simulink model "test_interconnect"  (Simulink 7.3)
settings: Solver=ode45  StartTime=0.0  StopTime=100  RelTol=1e-3
undefined symbols (not defined in the file): ROACH
libraries: xbsIndex_r4 x68, isi_correlator_lib x16, xps_library x7, casper_library x1
settings Model: Creator=wjm  LastModifiedBy=wjm
settings OptimizationCC: InitFltsAndDblsToZero=on

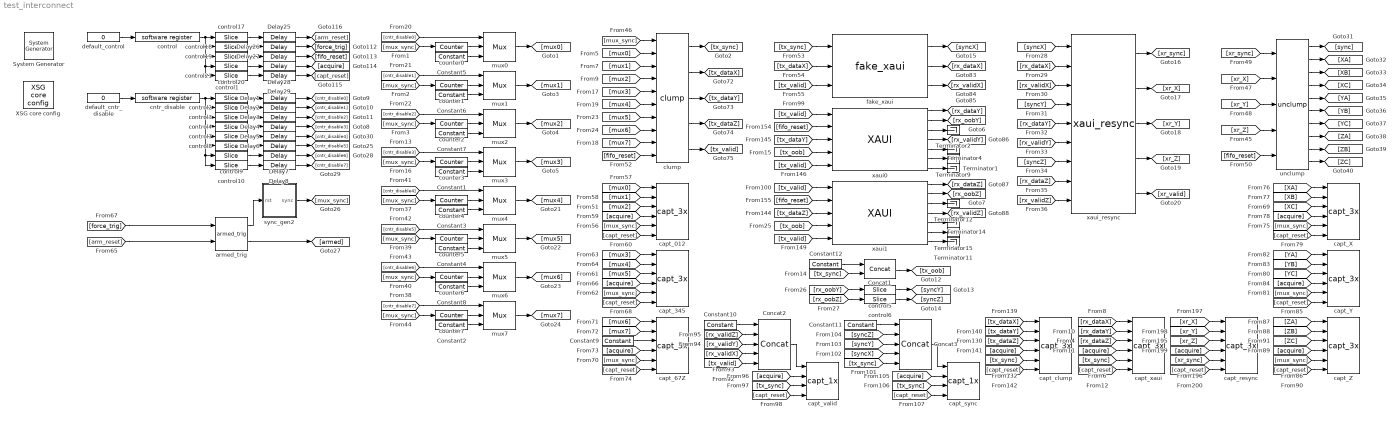
== system test_interconnect ==
  " System Generator" : xbsIndex_r4/ System Generator  Tag=genX  SystemSampleTime=-1  xilinxfamily=virtex5  part=xc5vsx95t  speed=-1  package=ff1136  synthesis_tool=XST  clock_wrapper=Clock Enables  directory=./test_interconnect/sysgen  testbench=off  simulink_period=1  sysclk_period=5  dcm_input_clock_period=100  incr_netlist=off  trim_vbits=Everywhere in SubSystem  dbl_ovrd=According to Block Masks  core_generation=According to Block Masks  run_coregen=off  deprecated_control=off  eval_field=0  block_type=sysgen
      settings: block_version=10.1.1
  Concat1 : xbsIndex_r4/Concat  num_inputs=2  dbl_ovrd=off  block_type=concat
      settings: block_version=11.3
  Concat2 : xbsIndex_r4/Concat  num_inputs=5  dbl_ovrd=off  block_type=concat
      settings: block_version=11.3
  Concat3 : xbsIndex_r4/Concat  num_inputs=5  dbl_ovrd=off  block_type=concat
      settings: block_version=11.3
  Constant{1..9} (9 alike) : xbsIndex_r4/Constant  arith_type=Unsigned  const=0  n_bits=8  bin_pt=0  explicit_period=on  period=1  equ=P=C  opselect=C  inp2=PCIN>>17  opr=+  inp1=P  carry=CIN  dbl_ovrd=off  block_type=constant
      settings: block_version=10.1.1
  Constant10 : xbsIndex_r4/Constant  arith_type=Unsigned  const=0  n_bits=28  bin_pt=0  explicit_period=on  period=1  equ=P=C  opselect=C  inp2=PCIN>>17  opr=+  inp1=P  carry=CIN  dbl_ovrd=off  block_type=constant
      settings: block_version=10.1.1
  Constant11 : xbsIndex_r4/Constant  arith_type=Unsigned  const=0  n_bits=28  bin_pt=0  explicit_period=on  period=1  equ=P=C  opselect=C  inp2=PCIN>>17  opr=+  inp1=P  carry=CIN  dbl_ovrd=off  block_type=constant
      settings: block_version=10.1.1
  Constant12 : xbsIndex_r4/Constant  arith_type=Unsigned  const=0  n_bits=3  bin_pt=0  explicit_period=on  period=1  equ=P=C  opselect=C  inp2=PCIN>>17  opr=+  inp1=P  carry=CIN  dbl_ovrd=off  block_type=constant
      settings: block_version=10.1.1
  Delay{1..8,25..29} (13 alike) : xbsIndex_r4/Delay  en=off  latency=3  dbl_ovrd=off  reg_retiming=off  block_type=delay
  Terminator{1..2,4,9,11..12,14..15} (8 alike) : Terminator
  XSG core config : xps_library/XSG core config  Tag=xps:xsg  SystemSampleTime=-1  hw_sys=ROACH:sx95t  ibob_linux=off  clk_src=sys_clk2x  iBOB_clk_src=sys_clk  BEE2_ctrl_clk_src=sys_clk  BEE2_usr_clk_src=sys_clk  ROACH_clk_src=sys_clk2x  CORR_clk_src=sys_clk  gpio_clk_io_group=iBOB:sma  gpio_clk_bit_index=0  clk_rate=200  sample_period=1  synthesis_tool=XST  mpc_type=powerpc440_ext
  armed_trig : isi_correlator_lib/armed_trig  SystemSampleTime=-1
  capt_012 : isi_correlator_lib/capt_3x  SystemSampleTime=-1
      link override bram0/convert_din: arith_type=Unsigned
      link override bram0/mem/sim_data_in: arith_type=Unsigned
      link override bram0/test_link_mux_demux_capt_demux_bram0_data_out: arith_type=Unsigned
      link override bram1/convert_din: arith_type=Unsigned
      link override bram1/mem/sim_data_in: arith_type=Unsigned
      link override bram1/test_link_mux_demux_capt_demux_bram1_data_out: arith_type=Unsigned
      link override bram2/convert_din: arith_type=Unsigned
      link override bram2/mem/sim_data_in: arith_type=Unsigned
      link override bram2/test_link_mux_demux_capt_demux_bram2_data_out: arith_type=Unsigned
  capt_345 : isi_correlator_lib/capt_3x  SystemSampleTime=-1
      link override bram0/convert_din: arith_type=Unsigned
      link override bram0/mem/sim_data_in: arith_type=Unsigned
      link override bram0/test_link_mux_demux_capt_demux_bram0_data_out: arith_type=Unsigned
      link override bram1/convert_din: arith_type=Unsigned
      link override bram1/mem/sim_data_in: arith_type=Unsigned
      link override bram1/test_link_mux_demux_capt_demux_bram1_data_out: arith_type=Unsigned
      link override bram2/convert_din: arith_type=Unsigned
      link override bram2/mem/sim_data_in: arith_type=Unsigned
      link override bram2/test_link_mux_demux_capt_demux_bram2_data_out: arith_type=Unsigned
  capt_67Z : isi_correlator_lib/capt_3x  SystemSampleTime=-1
      link override bram0/convert_din: arith_type=Unsigned
      link override bram0/mem/sim_data_in: arith_type=Unsigned
      link override bram0/test_link_mux_demux_capt_demux_bram0_data_out: arith_type=Unsigned
      link override bram1/convert_din: arith_type=Unsigned
      link override bram1/mem/sim_data_in: arith_type=Unsigned
      link override bram1/test_link_mux_demux_capt_demux_bram1_data_out: arith_type=Unsigned
      link override bram2/convert_din: arith_type=Unsigned
      link override bram2/mem/sim_data_in: arith_type=Unsigned
      link override bram2/test_link_mux_demux_capt_demux_bram2_data_out: arith_type=Unsigned
  capt_X : isi_correlator_lib/capt_3x  SystemSampleTime=-1
      link override bram0/convert_din: arith_type=Unsigned
      link override bram0/mem/sim_data_in: arith_type=Unsigned
      link override bram0/test_link_mux_demux_capt_demux_bram0_data_out: arith_type=Unsigned
      link override bram1/convert_din: arith_type=Unsigned
      link override bram1/mem/sim_data_in: arith_type=Unsigned
      link override bram1/test_link_mux_demux_capt_demux_bram1_data_out: arith_type=Unsigned
      link override bram2/convert_din: arith_type=Unsigned
      link override bram2/mem/sim_data_in: arith_type=Unsigned
      link override bram2/test_link_mux_demux_capt_demux_bram2_data_out: arith_type=Unsigned
  capt_Y : isi_correlator_lib/capt_3x  SystemSampleTime=-1
      link override bram0/convert_din: arith_type=Unsigned
      link override bram0/mem/sim_data_in: arith_type=Unsigned
      link override bram0/test_link_mux_demux_capt_demux_bram0_data_out: arith_type=Unsigned
      link override bram1/convert_din: arith_type=Unsigned
      link override bram1/mem/sim_data_in: arith_type=Unsigned
      link override bram1/test_link_mux_demux_capt_demux_bram1_data_out: arith_type=Unsigned
      link override bram2/convert_din: arith_type=Unsigned
      link override bram2/mem/sim_data_in: arith_type=Unsigned
      link override bram2/test_link_mux_demux_capt_demux_bram2_data_out: arith_type=Unsigned
  capt_Z : isi_correlator_lib/capt_3x  SystemSampleTime=-1
      link override bram0/convert_din: arith_type=Unsigned
      link override bram0/mem/sim_data_in: arith_type=Unsigned
      link override bram0/test_link_mux_demux_capt_demux_bram0_data_out: arith_type=Unsigned
      link override bram1/convert_din: arith_type=Unsigned
      link override bram1/mem/sim_data_in: arith_type=Unsigned
      link override bram1/test_link_mux_demux_capt_demux_bram1_data_out: arith_type=Unsigned
      link override bram2/convert_din: arith_type=Unsigned
      link override bram2/mem/sim_data_in: arith_type=Unsigned
      link override bram2/test_link_mux_demux_capt_demux_bram2_data_out: arith_type=Unsigned
  capt_clump : isi_correlator_lib/capt_3x  SystemSampleTime=-1
  capt_resync : isi_correlator_lib/capt_3x  SystemSampleTime=-1
      link override bram0/convert_din: arith_type=Unsigned
      link override bram0/mem/sim_data_in: arith_type=Unsigned
      link override bram0/test_link_mux_demux_capt_demux_bram0_data_out: arith_type=Unsigned
      link override bram1/convert_din: arith_type=Unsigned
      link override bram1/mem/sim_data_in: arith_type=Unsigned
      link override bram1/test_link_mux_demux_capt_demux_bram1_data_out: arith_type=Unsigned
      link override bram2/convert_din: arith_type=Unsigned
      link override bram2/mem/sim_data_in: arith_type=Unsigned
      link override bram2/test_link_mux_demux_capt_demux_bram2_data_out: arith_type=Unsigned
  capt_sync : isi_correlator_lib/capt_1x  SystemSampleTime=-1
  capt_valid : isi_correlator_lib/capt_1x  SystemSampleTime=-1
  capt_xaui : isi_correlator_lib/capt_3x  SystemSampleTime=-1
      link override bram0/convert_din: arith_type=Unsigned
      link override bram0/mem/sim_data_in: arith_type=Unsigned
      link override bram0/test_link_mux_demux_capt_demux_bram0_data_out: arith_type=Unsigned
      link override bram1/convert_din: arith_type=Unsigned
      link override bram1/mem/sim_data_in: arith_type=Unsigned
      link override bram1/test_link_mux_demux_capt_demux_bram1_data_out: arith_type=Unsigned
      link override bram2/convert_din: arith_type=Unsigned
      link override bram2/mem/sim_data_in: arith_type=Unsigned
      link override bram2/test_link_mux_demux_capt_demux_bram2_data_out: arith_type=Unsigned
  clump : isi_correlator_lib/clump  SystemSampleTime=-1  latency=1
  cntr_disable : xps_library/software register  Tag=xps:sw_reg  SystemSampleTime=-1  io_dir=From Processor  arith_type=Unsigned  bitwidth=32  bin_pt=0  sample_period=1  gw_name=test_interconnect_cntr_disable_user_data_out
      link override corr_3ghz_10_1_corr_id_user_data_out: arith_type=Unsigned  n_bits=32  bin_pt=0  period=1
      link override corr_3ghz_10_1_exp_corr_id_user_data_out: arith_type=Unsigned  n_bits=32  bin_pt=0  period=1
      link override isi_corr_eq_coeff_user_data_out: arith_type=Unsigned  n_bits=32  bin_pt=0  period=1
      link override isi_correlator_control_user_data_out: arith_type=Unsigned  n_bits=32  bin_pt=0  period=1
      link override isi_correlator_cropped_control_user_data_out: arith_type=Unsigned  n_bits=32  bin_pt=0  period=1
      link override isi_correlator_eq_coeff_user_data_out: arith_type=Unsigned  n_bits=32  bin_pt=0  period=1
      link override isi_spectrometer_control_user_data_out: arith_type=Unsigned  n_bits=32  bin_pt=0  period=1
      link override isi_spectrometer_cropped_control_user_data_out: arith_type=Unsigned  n_bits=32  bin_pt=0  period=1
      link override isi_spectrometer_with_pfb_control_user_data_out: arith_type=Unsigned  n_bits=32  bin_pt=0  period=1
      link override roach_spectrometer_control_user_data_out: arith_type=Unsigned  n_bits=32  bin_pt=0  period=1
      link override test_link_mux_demux_control_user_data_out: arith_type=Unsigned  n_bits=32  bin_pt=0  period=1
  control : xps_library/software register  Tag=xps:sw_reg  SystemSampleTime=-1  io_dir=From Processor  arith_type=Unsigned  bitwidth=32  bin_pt=0  sample_period=1  gw_name=test_interconnect_control_user_data_out
      link override corr_3ghz_10_1_corr_id_user_data_out: arith_type=Unsigned  n_bits=32  bin_pt=0  period=1
      link override corr_3ghz_10_1_exp_corr_id_user_data_out: arith_type=Unsigned  n_bits=32  bin_pt=0  period=1
      link override isi_corr_eq_coeff_user_data_out: arith_type=Unsigned  n_bits=32  bin_pt=0  period=1
      link override isi_correlator_control_user_data_out: arith_type=Unsigned  n_bits=32  bin_pt=0  period=1
      link override isi_correlator_cropped_control_user_data_out: arith_type=Unsigned  n_bits=32  bin_pt=0  period=1
      link override isi_correlator_eq_coeff_user_data_out: arith_type=Unsigned  n_bits=32  bin_pt=0  period=1
      link override isi_spectrometer_control_user_data_out: arith_type=Unsigned  n_bits=32  bin_pt=0  period=1
      link override isi_spectrometer_cropped_control_user_data_out: arith_type=Unsigned  n_bits=32  bin_pt=0  period=1
      link override isi_spectrometer_with_pfb_control_user_data_out: arith_type=Unsigned  n_bits=32  bin_pt=0  period=1
      link override roach_spectrometer_control_user_data_out: arith_type=Unsigned  n_bits=32  bin_pt=0  period=1
      link override test_link_mux_demux_control_user_data_out: arith_type=Unsigned  n_bits=32  bin_pt=0  period=1
  control1 : xbsIndex_r4/Slice  nbits=1  boolean_output=off  mode=Lower Bit Location + Width  bit1=0  base1=MSB of Input  bit0=0  base0=LSB of Input  dbl_ovrd=off  block_type=slice
      settings: block_version=10.1.3
  control10 : xbsIndex_r4/Slice  nbits=1  boolean_output=off  mode=Lower Bit Location + Width  bit1=0  base1=MSB of Input  bit0=7  base0=LSB of Input  dbl_ovrd=off  block_type=slice
      settings: block_version=10.1.3
  control17 : xbsIndex_r4/Slice  nbits=1  boolean_output=on  mode=Lower Bit Location + Width  bit1=0  base1=MSB of Input  bit0=0  base0=LSB of Input  dbl_ovrd=off  block_type=slice
      settings: infoedit="Extracts a given range of bits from each input sample and presents it at the output.  The output type is ordinarily unsigned with binary point at zero, but can be Boolean when the slice is one bit wide.<P><P>Hardware notes: In hardware this block costs nothing."  block_version=10.1.3
  control18 : xbsIndex_r4/Slice  nbits=1  boolean_output=on  mode=Lower Bit Location + Width  bit1=0  base1=MSB of Input  bit0=1  base0=LSB of Input  dbl_ovrd=off  block_type=slice
      settings: infoedit="Extracts a given range of bits from each input sample and presents it at the output.  The output type is ordinarily unsigned with binary point at zero, but can be Boolean when the slice is one bit wide.<P><P>Hardware notes: In hardware this block costs nothing."  block_version=10.1.3
  control19 : xbsIndex_r4/Slice  nbits=1  boolean_output=on  mode=Lower Bit Location + Width  bit1=0  base1=MSB of Input  bit0=2  base0=LSB of Input  dbl_ovrd=off  block_type=slice
      settings: infoedit="Extracts a given range of bits from each input sample and presents it at the output.  The output type is ordinarily unsigned with binary point at zero, but can be Boolean when the slice is one bit wide.<P><P>Hardware notes: In hardware this block costs nothing."  block_version=10.1.3
  control2 : xbsIndex_r4/Slice  nbits=1  boolean_output=off  mode=Lower Bit Location + Width  bit1=0  base1=MSB of Input  bit0=1  base0=LSB of Input  dbl_ovrd=off  block_type=slice
      settings: block_version=10.1.3
  control20 : xbsIndex_r4/Slice  nbits=1  boolean_output=on  mode=Lower Bit Location + Width  bit1=0  base1=MSB of Input  bit0=3  base0=LSB of Input  dbl_ovrd=off  block_type=slice
      settings: infoedit="Extracts a given range of bits from each input sample and presents it at the output.  The output type is ordinarily unsigned with binary point at zero, but can be Boolean when the slice is one bit wide.<P><P>Hardware notes: In hardware this block costs nothing."  block_version=10.1.3
  control21 : xbsIndex_r4/Slice  nbits=1  boolean_output=on  mode=Lower Bit Location + Width  bit1=0  base1=MSB of Input  bit0=4  base0=LSB of Input  dbl_ovrd=off  block_type=slice
      settings: infoedit="Extracts a given range of bits from each input sample and presents it at the output.  The output type is ordinarily unsigned with binary point at zero, but can be Boolean when the slice is one bit wide.<P><P>Hardware notes: In hardware this block costs nothing."  block_version=10.1.3
  control3 : xbsIndex_r4/Slice  nbits=1  boolean_output=off  mode=Lower Bit Location + Width  bit1=0  base1=MSB of Input  bit0=2  base0=LSB of Input  dbl_ovrd=off  block_type=slice
      settings: block_version=10.1.3
  control4 : xbsIndex_r4/Slice  nbits=1  boolean_output=off  mode=Lower Bit Location + Width  bit1=0  base1=MSB of Input  bit0=3  base0=LSB of Input  dbl_ovrd=off  block_type=slice
      settings: block_version=10.1.3
  control5 : xbsIndex_r4/Slice  nbits=1  boolean_output=on  mode=Lower Bit Location + Width  bit1=0  base1=MSB of Input  bit0=0  base0=LSB of Input  dbl_ovrd=off  block_type=slice
      settings: infoedit="Extracts a given range of bits from each input sample and presents it at the output.  The output type is ordinarily unsigned with binary point at zero, but can be Boolean when the slice is one bit wide.<P><P>Hardware notes: In hardware this block costs nothing."  block_version=10.1.3
  control6 : xbsIndex_r4/Slice  nbits=1  boolean_output=on  mode=Lower Bit Location + Width  bit1=0  base1=MSB of Input  bit0=0  base0=LSB of Input  dbl_ovrd=off  block_type=slice
      settings: infoedit="Extracts a given range of bits from each input sample and presents it at the output.  The output type is ordinarily unsigned with binary point at zero, but can be Boolean when the slice is one bit wide.<P><P>Hardware notes: In hardware this block costs nothing."  block_version=10.1.3
  control7 : xbsIndex_r4/Slice  nbits=1  boolean_output=off  mode=Lower Bit Location + Width  bit1=0  base1=MSB of Input  bit0=4  base0=LSB of Input  dbl_ovrd=off  block_type=slice
      settings: block_version=10.1.3
  control8 : xbsIndex_r4/Slice  nbits=1  boolean_output=off  mode=Lower Bit Location + Width  bit1=0  base1=MSB of Input  bit0=5  base0=LSB of Input  dbl_ovrd=off  block_type=slice
      settings: block_version=10.1.3
  control9 : xbsIndex_r4/Slice  nbits=1  boolean_output=off  mode=Lower Bit Location + Width  bit1=0  base1=MSB of Input  bit0=6  base0=LSB of Input  dbl_ovrd=off  block_type=slice
      settings: block_version=10.1.3
  counter0 : xbsIndex_r4/Counter  cnt_type=Free Running  cnt_to=Inf  operation=Up  start_count=0  cnt_by_val=128  arith_type=Unsigned  n_bits=8  bin_pt=0  load_pin=off  rst=on  en=off  explicit_period=on  period=1  dbl_ovrd=off  use_behavioral_HDL=off  implementation=Fabric  use_rpm=off  block_type=counter
  counter1 : xbsIndex_r4/Counter  cnt_type=Free Running  cnt_to=Inf  operation=Up  start_count=0  cnt_by_val=64  arith_type=Unsigned  n_bits=8  bin_pt=0  load_pin=off  rst=on  en=off  explicit_period=on  period=1  dbl_ovrd=off  use_behavioral_HDL=off  implementation=Fabric  use_rpm=off  block_type=counter
  counter2 : xbsIndex_r4/Counter  cnt_type=Free Running  cnt_to=Inf  operation=Up  start_count=0  cnt_by_val=32  arith_type=Unsigned  n_bits=8  bin_pt=0  load_pin=off  rst=on  en=off  explicit_period=on  period=1  dbl_ovrd=off  use_behavioral_HDL=off  implementation=Fabric  use_rpm=off  block_type=counter
  counter3 : xbsIndex_r4/Counter  cnt_type=Free Running  cnt_to=Inf  operation=Up  start_count=0  cnt_by_val=16  arith_type=Unsigned  n_bits=8  bin_pt=0  load_pin=off  rst=on  en=off  explicit_period=on  period=1  dbl_ovrd=off  use_behavioral_HDL=off  implementation=Fabric  use_rpm=off  block_type=counter
  counter4 : xbsIndex_r4/Counter  cnt_type=Free Running  cnt_to=Inf  operation=Up  start_count=0  cnt_by_val=8  arith_type=Unsigned  n_bits=8  bin_pt=0  load_pin=off  rst=on  en=off  explicit_period=on  period=1  dbl_ovrd=off  use_behavioral_HDL=off  implementation=Fabric  use_rpm=off  block_type=counter
  counter5 : xbsIndex_r4/Counter  cnt_type=Free Running  cnt_to=Inf  operation=Up  start_count=0  cnt_by_val=4  arith_type=Unsigned  n_bits=8  bin_pt=0  load_pin=off  rst=on  en=off  explicit_period=on  period=1  dbl_ovrd=off  use_behavioral_HDL=off  implementation=Fabric  use_rpm=off  block_type=counter
  counter6 : xbsIndex_r4/Counter  cnt_type=Free Running  cnt_to=Inf  operation=Up  start_count=0  cnt_by_val=2  arith_type=Unsigned  n_bits=8  bin_pt=0  load_pin=off  rst=on  en=off  explicit_period=on  period=1  dbl_ovrd=off  use_behavioral_HDL=off  implementation=Fabric  use_rpm=off  block_type=counter
  counter7 : xbsIndex_r4/Counter  cnt_type=Free Running  cnt_to=Inf  operation=Up  start_count=0  cnt_by_val=1  arith_type=Unsigned  n_bits=8  bin_pt=0  load_pin=off  rst=on  en=off  explicit_period=on  period=1  dbl_ovrd=off  use_behavioral_HDL=off  implementation=Fabric  use_rpm=off  block_type=counter
  default_cntr_disable : Constant  Value=0  OutDataType=sfix(16)  OutScaling=2^0  SampleTime=1
  default_control : Constant  Value=0  OutDataType=sfix(16)  OutScaling=2^0  SampleTime=1
  fake_xaui : isi_correlator_lib/fake_xaui  SystemSampleTime=-1  latency=32
  mux{0..7} (8 alike) : xbsIndex_r4/Mux  inputs=2  en=off  latency=0  precision=Full  arith_type=Unsigned  n_bits=16  bin_pt=14  quantization=Truncate  overflow=Wrap  dbl_ovrd=off  block_type=mux
      settings: block_version=11.3
  sync_gen2 : Subsystem  AncestorBlock=isi_correlator_lib/sync_gen2  mask(sync_gen2){using_pfb_fir=off, pfb_fir_taps=4, using_fft=off, fft_size=7, fft_inputs=4, fft_orders=[2 2 2 1], using_ct=off, ct_type=Double-buffered, using_vacc=off, vacc_length=0, using_scale_factor=on, scale_factor=2^10}
      mask prompts: using_pfb_fir "This design uses a PFB FIR."; pfb_fir_taps "Number of taps in PFB FIR:"; using_fft "This design uses an FFT."; fft_size "Size of FFT: (2^?)"; fft_inputs "Number of FFT inputs: (2^?)"; fft_orders "Order of FFT reorders: (vector)"; using_ct "This design uses a corner turner."; ct_type "Type of reorder operation:"; using_vacc "This design uses a vector accumulator."; vacc_length "Length of accumulations: (2^?)"; using_scale_factor "Scale the minimum period by an arbitrary amount."; scale_factor "Scale factor:"
      mask help: This block generates a sync pulse of an appropriate period based on the specified mask parameters.
      mask init:
      | sync_gen2_init(gcb, ...
      |     'using_pfb_fir', using_pfb_fir, ...
      |     'pfb_fir_taps', pfb_fir_taps, ...
      |     'using_fft', using_fft, ...
      |     'fft_size', fft_size, ...
      |     'fft_inputs', fft_inputs, ...
      |     'fft_orders', fft_orders, ...
      |     'using_ct', using_ct, ...
      |     'ct_type', ct_type, ...
      |     'using_vacc', using_vacc, ...
      |     'vacc_length', vacc_length, ...
      |     'using_scale_factor', using_scale_factor, ...
      |     'scale_factor', scale_factor);
      settings: AttributesFormatString=sync_period=1024
      mask StyleString: checkbox,edit,checkbox,edit,edit,edit,checkbox,popup(Double-buffered|In-place),checkbox,edit,checkbox,edit
      mask CallbackString:
      | thisVariable = 'using_pfb_fir';
      | affectedVars = {'pfb_fir_taps'};
      | 
      | thisBlock = gcb();
      | thisVarState = get_param(thisBlock, thisVariable);
      | maskNames = get_param(thisBlock, 'MaskNames');
      | maskEnables = get_param(thisBlock, 'MaskEnables');
      | 
      | for varName = affectedVars
      |     varIndex = find(ismember(maskNames, varName));
      |     maskEnables{varIndex} = thisVarState;
      | end
      | 
      | set_param(thisBlock, 'MaskEnables', maskEnables);||thisVariable = 'using_fft';
      | affectedVars = {'fft_size', 'fft_inputs', 'fft_orders'};
      | 
      | thisBlock = gcb();
      | thisVarState = get_param(thisBlock, thisVariable);
      | maskNames = get_param(thisBlock, 'MaskNames');
      | maskEnables = get_param(thisBlock, 'MaskEnables');
      | 
      | for varName = affectedVars
      |     varIndex = find(ismember(maskNames, varName));
      |     maskEnables{varIndex} = thisVarState;
      | end
      | 
      | set_param(thisBlock, 'MaskEnables', maskEnables);||||thisVariable = 'using_ct';
      | affectedVars = {'ct_type'};
      | 
      | thisBlock = gcb();
      | thisVarState = get_param(thisBlock, thisVariable);
      | maskNames = get_param(thisBlock, 'MaskNames');
      | maskEnables = get_param(thisBlock, 'MaskEnables');
      | 
      | for varName = affectedVars
      |     varIndex = find(ismember(maskNames, varName));
      |     maskEnables{varIndex} = thisVarState;
      | end
      | 
      | set_param(thisBlock, 'MaskEnables', maskEnables);||thisVariable = 'using_vacc';
      | affectedVars = {'vacc_length'};
      | 
      | thisBlock = gcb();
      | thisVarState = get_param(thisBlock, thisVariable);
      | maskNames = get_param(thisBlock, 'MaskNames');
      | maskEnables = get_param(thisBlock, 'MaskEnables');
      | 
      | for varName = affectedVars
      |     varIndex = find(ismember(maskNames, varName));
      |     maskEnables{varIndex} = thisVarState;
      | end
      | 
      | set_param(thisBlock, 'MaskEnables', maskEnables);||thisVariable = 'using_scale_factor';
      | affectedVars = {'scale_factor'};
      | 
      | thisBlock = gcb();
      | thisVarState = get_param(thisBlock, thisVariable);
      | maskNames = get_param(thisBlock, 'MaskNames');
      | maskEnables = get_param(thisBlock, 'MaskEnables');
      | 
      | for varName = affectedVars
      |     varIndex = find(ismember(maskNames, varName));
      |     maskEnables{varIndex} = thisVarState;
      | end
      | 
      | set_param(thisBlock, 'MaskEnables', maskEnables);|
  unclump : isi_correlator_lib/unclump  SystemSampleTime=-1  latency=1
  xaui0 : xps_library/XAUI  Tag=xps:xaui  SystemSampleTime=-1  demux=2  port=ROACH:0  open_phy=on  show_param=off  pre_emph=3  swing=800
      link override convert_tx_data: n_bits=32
      link override convert_tx_outofband: n_bits=4
      link override test_link_mux_demux_xaui0_rx_data: n_bits=32
      link override test_link_mux_demux_xaui0_rx_outofband: n_bits=4
  xaui1 : xps_library/XAUI  Tag=xps:xaui  SystemSampleTime=-1  demux=2  port=ROACH:1  open_phy=on  show_param=off  pre_emph=3  swing=800
      link override convert_tx_data: n_bits=32
      link override convert_tx_outofband: n_bits=4
      link override test_link_mux_demux_xaui1_rx_data: n_bits=32
      link override test_link_mux_demux_xaui1_rx_outofband: n_bits=4
  xaui_resync : isi_correlator_lib/xaui_resync  SystemSampleTime=-1  buffer_depth=8  logic_latency=1
  wires:
  [tx_dataX] -> capt_clump/1
  [tx_dataY] -> capt_clump/2
  [tx_dataZ] -> capt_clump/3
  [capt_reset] -> capt_clump/6
  [tx_sync] -> fake_xaui/1
  [tx_dataX] -> fake_xaui/2
  [tx_valid] -> fake_xaui/3
  [fifo_reset] -> xaui0/2
  [tx_dataY] -> xaui0/3
  [tx_valid] -> xaui0/5
  [fifo_reset] -> xaui1/2
  [tx_dataZ] -> xaui1/3
  [tx_oob] -> xaui1/4
  [tx_valid] -> xaui1/5
  xaui0/1 -> [rx_dataY]
  xaui0/2 -> [rx_oobY]
  xaui0/3 -> Terminator2/1
  xaui0/4 -> [rx_validY]
  xaui0/5 -> Terminator4/1
  xaui0/6 -> Terminator9/1
  xaui0/7 -> Terminator1/1
  xaui1/1 -> [rx_dataZ]
  xaui1/2 -> [rx_oobZ]
  xaui1/3 -> Terminator12/1
  xaui1/4 -> [rx_validZ]
  xaui1/5 -> Terminator14/1
  xaui1/6 -> Terminator15/1
  xaui1/7 -> Terminator11/1
  fake_xaui/2 -> [rx_dataX]
  fake_xaui/3 -> [rx_validX]
  [acquire] -> capt_clump/4
  [tx_sync] -> capt_clump/5
  fake_xaui/1 -> [syncX]
  [xr_Y] -> capt_resync/2
  [xr_Z] -> capt_resync/3
  [capt_reset] -> capt_resync/6
  [acquire] -> capt_resync/4
  [xr_sync] -> capt_resync/5
  [arm_reset] -> armed_trig/2
  [force_trig] -> armed_trig/1
  armed_trig/1 -> sync_gen2/1(rst)
  armed_trig/2 -> [armed]
  sync_gen2/1(sync) -> [mux_sync]
  control21/1 -> Delay29/1
  control20/1 -> Delay28/1
  control19/1 -> Delay27/1
  control18/1 -> Delay26/1
  control17/1 -> Delay25/1
  control/1 -> control17/1, control18/1, control19/1, control21/1, control20/1
  Delay26/1 -> [force_trig]
  Delay27/1 -> [fifo_reset]
  Delay28/1 -> [acquire]
  Delay29/1 -> [capt_reset]
  default_control/1 -> control/1
  Delay25/1 -> [arm_reset]
  [xr_X] -> capt_resync/1
  [mux_sync] -> counter0/1
  [mux_sync] -> counter1/1
  [mux_sync] -> counter2/1
  [rx_dataY] -> capt_xaui/2
  [rx_dataZ] -> capt_xaui/3
  [capt_reset] -> capt_xaui/6
  [acquire] -> capt_xaui/4
  [tx_sync] -> capt_xaui/5
  [rx_dataX] -> capt_xaui/1
  [tx_valid] -> xaui0/1
  [tx_valid] -> xaui1/1
  mux0/1 -> [mux0]
  mux1/1 -> [mux1]
  mux2/1 -> [mux2]
  counter2/1 -> mux2/2
  Constant7/1 -> mux2/3
  Constant6/1 -> mux1/3
  counter1/1 -> mux1/2
  Constant5/1 -> mux0/3
  counter0/1 -> mux0/2
  [cntr_disable0] -> mux0/1
  [cntr_disable1] -> mux1/1
  [cntr_disable2] -> mux2/1
  default_cntr_disable/1 -> cntr_disable/1
  cntr_disable/1 -> control1/1, control2/1, control3/1, control4/1, control7/1, control8/1, control10/1, control9/1
  control1/1 -> Delay1/1
  Delay1/1 -> [cntr_disable0]
  control2/1 -> Delay2/1
  Delay2/1 -> [cntr_disable1]
  control3/1 -> Delay3/1
  Delay3/1 -> [cntr_disable2]
  [mux_sync] -> counter3/1
  mux3/1 -> [mux3]
  counter3/1 -> mux3/2
  Constant1/1 -> mux3/3
  [cntr_disable3] -> mux3/1
  control4/1 -> Delay4/1
  Delay4/1 -> [cntr_disable3]
  [mux_sync] -> clump/1
  [mux0] -> clump/2
  [mux1] -> clump/3
  [mux2] -> clump/4
  [mux3] -> clump/5
  [mux4] -> clump/6
  [mux5] -> clump/7
  [mux6] -> clump/8
  [mux7] -> clump/9
  [fifo_reset] -> clump/10
  clump/1 -> [tx_sync]
  clump/2 -> [tx_dataX]
  clump/3 -> [tx_dataY]
  clump/4 -> [tx_dataZ]
  clump/5 -> [tx_valid]
  Concat1/1 -> [tx_oob]
  Constant12/1 -> Concat1/1
  [tx_sync] -> Concat1/2
  [tx_oob] -> xaui0/4
  [rx_oobZ] -> control6/1
  [rx_oobY] -> control5/1
  control5/1 -> [syncY]
  control6/1 -> [syncZ]
  [syncX] -> xaui_resync/1
  [rx_dataX] -> xaui_resync/2
  [rx_validX] -> xaui_resync/3
  [syncY] -> xaui_resync/4
  [rx_dataY] -> xaui_resync/5
  [rx_validY] -> xaui_resync/6
  [syncZ] -> xaui_resync/7
  [rx_dataZ] -> xaui_resync/8
  [rx_validZ] -> xaui_resync/9
  xaui_resync/1 -> [xr_sync]
  xaui_resync/2 -> [xr_X]
  xaui_resync/3 -> [xr_Y]
  xaui_resync/4 -> [xr_Z]
  xaui_resync/5 -> [xr_valid]
  [mux_sync] -> counter4/1
  [mux_sync] -> counter5/1
  [mux_sync] -> counter6/1
  mux4/1 -> [mux4]
  mux5/1 -> [mux5]
  mux6/1 -> [mux6]
  counter6/1 -> mux6/2
  Constant8/1 -> mux6/3
  Constant4/1 -> mux5/3
  counter5/1 -> mux5/2
  Constant3/1 -> mux4/3
  counter4/1 -> mux4/2
  [cntr_disable4] -> mux4/1
  [cntr_disable5] -> mux5/1
  [cntr_disable6] -> mux6/1
  [mux_sync] -> counter7/1
  mux7/1 -> [mux7]
  counter7/1 -> mux7/2
  Constant2/1 -> mux7/3
  [cntr_disable7] -> mux7/1
  control7/1 -> Delay5/1
  Delay5/1 -> [cntr_disable4]
  control8/1 -> Delay6/1
  Delay6/1 -> [cntr_disable5]
  control9/1 -> Delay7/1
  Delay7/1 -> [cntr_disable6]
  control10/1 -> Delay8/1
  Delay8/1 -> [cntr_disable7]
  [xr_sync] -> unclump/1
  [xr_X] -> unclump/2
  [xr_Y] -> unclump/3
  [xr_Z] -> unclump/4
  [fifo_reset] -> unclump/5
  unclump/1 -> [sync]
  unclump/2 -> [XA]
  unclump/3 -> [XB]
  unclump/4 -> [XC]
  unclump/5 -> [YA]
  unclump/6 -> [YB]
  unclump/7 -> [YC]
  unclump/8 -> [ZA]
  unclump/9 -> [ZB]
  unclump/10 -> [ZC]
  [mux1] -> capt_012/2
  [mux2] -> capt_012/3
  [capt_reset] -> capt_012/6
  [acquire] -> capt_012/4
  [mux_sync] -> capt_012/5
  [mux0] -> capt_012/1
  [mux4] -> capt_345/2
  [mux5] -> capt_345/3
  [capt_reset] -> capt_345/6
  [acquire] -> capt_345/4
  [mux_sync] -> capt_345/5
  [mux3] -> capt_345/1
  [mux7] -> capt_67Z/2
  Constant9/1 -> capt_67Z/3
  [capt_reset] -> capt_67Z/6
  [acquire] -> capt_67Z/4
  [mux_sync] -> capt_67Z/5
  [mux6] -> capt_67Z/1
  [XB] -> capt_X/2
  [XC] -> capt_X/3
  [capt_reset] -> capt_X/6
  [acquire] -> capt_X/4
  [mux_sync] -> capt_X/5
  [XA] -> capt_X/1
  [YB] -> capt_Y/2
  [YC] -> capt_Y/3
  [capt_reset] -> capt_Y/6
  [acquire] -> capt_Y/4
  [mux_sync] -> capt_Y/5
  [YA] -> capt_Y/1
  [ZB] -> capt_Z/2
  [capt_reset] -> capt_Z/6
  [acquire] -> capt_Z/4
  [mux_sync] -> capt_Z/5
  [ZA] -> capt_Z/1
  [ZC] -> capt_Z/3
  Concat2/1 -> capt_valid/1
  [acquire] -> capt_valid/2
  [tx_sync] -> capt_valid/3
  [capt_reset] -> capt_valid/4
  Constant10/1 -> Concat2/1
  [rx_validZ] -> Concat2/2
  [rx_validY] -> Concat2/3
  [rx_validX] -> Concat2/4
  [tx_valid] -> Concat2/5
  Concat3/1 -> capt_sync/1
  [acquire] -> capt_sync/2
  [tx_sync] -> capt_sync/3
  [capt_reset] -> capt_sync/4
  Constant11/1 -> Concat3/1
  [syncZ] -> Concat3/2
  [syncY] -> Concat3/3
  [syncX] -> Concat3/4
  [tx_sync] -> Concat3/5

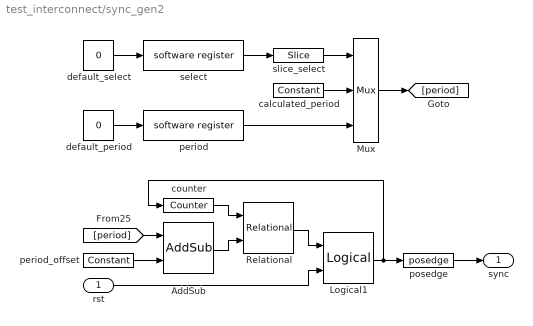
== system test_interconnect/sync_gen2 ==
  rst : Inport  OutDataType=sfix(16)  OutScaling=2^0
  AddSub : xbsIndex_r4/AddSub  mode=Subtraction  use_carryin=off  use_carryout=off  en=off  latency=2  precision=Full  arith_type=Unsigned  n_bits=16  bin_pt=14  quantization=Truncate  overflow=Wrap  dbl_ovrd=off  use_behavioral_HDL=off  hw_selection=Fabric  pipelined=off  use_rpm=on  block_type=addsub
      settings: block_version=10.1.3
  Logical1 : xbsIndex_r4/Logical  logical_function=OR  inputs=2  en=off  latency=0  precision=Full  arith_type=Unsigned  n_bits=16  bin_pt=0  align_bp=on  dbl_ovrd=off  block_type=logical
  Mux : xbsIndex_r4/Mux  inputs=2  en=off  latency=0  precision=Full  arith_type=Unsigned  n_bits=16  bin_pt=14  quantization=Truncate  overflow=Wrap  dbl_ovrd=off  block_type=mux
  Relational : xbsIndex_r4/Relational  mode=a>=b  en=off  latency=1  dbl_ovrd=off  block_type=relational
      settings: block_version=10.1.3
  calculated_period : xbsIndex_r4/Constant  arith_type=Unsigned  const=1024  n_bits=32  bin_pt=0  explicit_period=on  period=1  equ=P=C  opselect=C  inp2=PCIN>>17  opr=+  inp1=P  carry=CIN  dbl_ovrd=off  block_type=constant
      settings: block_version=10.1.1
  counter : xbsIndex_r4/Counter  cnt_type=Free Running  cnt_to=Inf  operation=Up  start_count=0  cnt_by_val=1  arith_type=Unsigned  n_bits=32  bin_pt=0  load_pin=off  rst=on  en=off  explicit_period=on  period=1  dbl_ovrd=off  use_behavioral_HDL=off  implementation=Fabric  use_rpm=off  block_type=counter
  default_period : Constant  Value=0  OutDataType=sfix(16)  OutScaling=2^0  SampleTime=1
  default_select : Constant  Value=0  OutDataType=sfix(16)  OutScaling=2^0  SampleTime=1
  period : xps_library/software register  Tag=xps:sw_reg  SystemSampleTime=-1  io_dir=From Processor  arith_type=Unsigned  bitwidth=32  bin_pt=0  sample_period=1  gw_name=test_interconnect_sync_gen2_period_user_data_out
      link override test_link_mux_demux_sync_gen2_period_user_data_out: arith_type=Unsigned  n_bits=32  bin_pt=0  period=1
  period_offset : xbsIndex_r4/Constant  arith_type=Unsigned  const=3  n_bits=32  bin_pt=0  explicit_period=on  period=1  equ=P=C  opselect=C  inp2=PCIN>>17  opr=+  inp1=P  carry=CIN  dbl_ovrd=off  block_type=constant
      settings: block_version=10.1.1
  posedge : casper_library/Misc/posedge  Tag=Rising Edge Detector  SystemSampleTime=-1
  select : xps_library/software register  Tag=xps:sw_reg  SystemSampleTime=-1  io_dir=From Processor  arith_type=Unsigned  bitwidth=32  bin_pt=0  sample_period=1  gw_name=test_interconnect_sync_gen2_select_user_data_out
      link override test_link_mux_demux_sync_gen2_select_user_data_out: arith_type=Unsigned  n_bits=32  bin_pt=0  period=1
  slice_select : xbsIndex_r4/Slice  nbits=1  boolean_output=on  mode=Lower Bit Location + Width  bit1=0  base1=MSB of Input  bit0=0  base0=LSB of Input  dbl_ovrd=off  block_type=slice
      settings: infoedit="Extracts a given range of bits from each input sample and presents it at the output.  The output type is ordinarily unsigned with binary point at zero, but can be Boolean when the slice is one bit wide.<P><P>Hardware notes: In hardware this block costs nothing."  block_version=10.1.3
  sync : Outport  OutDataType=sfix(16)  OutScaling=2^0
  wires:
  Mux/1 -> [period]
  period/1 -> Mux/3
  calculated_period/1 -> Mux/2
  slice_select/1 -> Mux/1
  default_period/1 -> period/1
  select/1 -> slice_select/1
  default_select/1 -> select/1
  [period] -> AddSub/1
  period_offset/1 -> AddSub/2
  AddSub/1 -> Relational/2
  counter/1 -> Relational/1
  Logical1/1 -> posedge/1, counter/1
  posedge/1 -> sync/1
  Relational/1 -> Logical1/1
  rst/1 -> Logical1/2
